simulink model "Tipo1Normalito"  (R2021b)
settings: Solver=VariableStepAuto  StartTime=0.0  StopTime=10.0  RelTol=1e-3
settings Model: Creator=Andre  LastModifiedBy=Andre

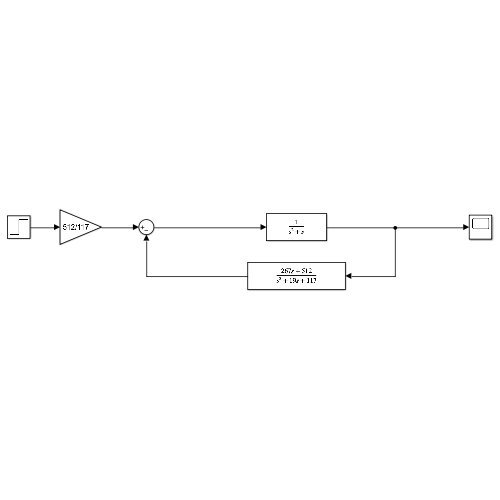
[thumbnail: Simulink's stored preview of the top-level diagram]
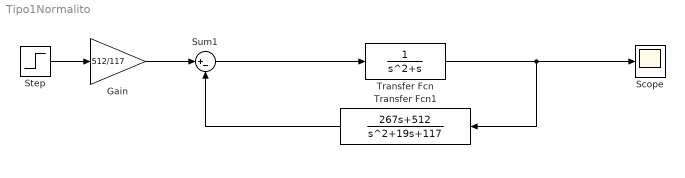
== system Tipo1Normalito ==
  Gain : Gain  Gain=512/117
  Scope : Scope
  Step : Step  Time=0  SampleTime=0
  Sum1 : Sum  Inputs=|+-
  Transfer Fcn : TransferFcn  Numerator=[0 0 1]  Denominator=[1 1 0]
  Transfer Fcn1 : TransferFcn  Numerator=[0 267 512]  Denominator=[1 19 117]
  wires:
  Sum1/1 -> Transfer Fcn/1
  Transfer Fcn/1 -> Transfer Fcn1/1, Scope/1
  Step/1 -> Gain/1
  Gain/1 -> Sum1/1
  Transfer Fcn1/1 -> Sum1/2
